simulink model "HighRangeSensor"  (R2016a)
settings: Solver=FixedStepAuto  StartTime=0.0  StopTime=10.0  FixedStep=0.1  RelTol=1e-3
settings Model: Creator=Josef  LastModifiedBy=Josef
settings GRTTargetCC: GeneratePreprocessorConditionals=Use local settings

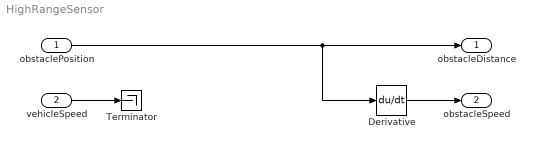
== system HighRangeSensor ==
  obstaclePosition : Inport
      settings: AttributesFormatString=signal
  vehicleSpeed : Inport  Port=2
      settings: AttributesFormatString=speed
  Derivative : Derivative
  Terminator : Terminator
  obstacleDistance : Outport
      settings: AttributesFormatString=distance
  obstacleSpeed : Outport  Port=2
      settings: AttributesFormatString=speed
  wires:
  obstaclePosition/1 -> Derivative/1, obstacleDistance/1
  vehicleSpeed/1 -> Terminator/1
  Derivative/1 -> obstacleSpeed/1
